simulink model "Controllo_XY"  (R2020b)
settings: Solver=VariableStepAuto  StartTime=0.0  StopTime=3  RelTol=1e-3
values from neighbouring files (symbols this model uses):
  mx = config_dc_x(parx)    [Main_Strategia_di_pilotaggio.m]    (also in Main_traiettoria.m; Main_traiettoria_ordinato.m)
  my = config_dc_y(pary)    [Main_Strategia_di_pilotaggio.m]    (also in Main_traiettoria.m; Main_traiettoria_ordinato.m)
undefined symbols (not defined in the file or in its folder): accelerazioni, accelerazioniy, Evaluate_Trajectory, parx, pary
libraries: cstblocks x8
settings Model: Creator=stefa  LastModifiedBy=user
settings DebuggingCC: SFMachineParentedDataDiag=error

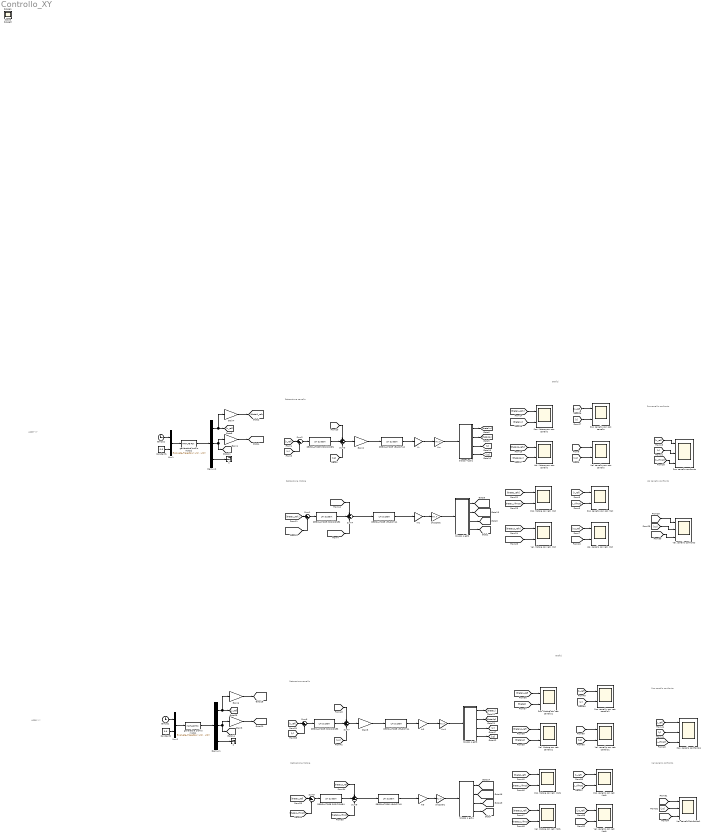
== system Controllo_XY ==
  note: ASSE "X"
  note: Retroazione carrello
  note: Retroazione Motore
  note: Grafici
  note: Pos carrello confronto
  note: Vel carrello confronto
  note: Retroazione carrello
  note: Grafici
  note: Retroazione Motore
  note: Pos carrello confronto
  note: Vel carrello confronto
  note: ASSE "Y"
  " 1" : Terminator
  " 2" : Terminator
  Constant1 : Constant  Value=0.6
  Constant2 : Constant  Value=0.6
  Demux1 : Demux  Outputs=3
  Demux2 : Demux  Outputs=3
  Gain1 : Gain  Gain=1/parx.tau
  Gain2 : Gain  Gain=1/parx.tau
  Gain3 : Gain  Gain=1/pary.tau
  Gain4 : Gain  Gain=1/parx.tau
  Gain5 : Gain  Gain=1/pary.tau
  Gain6 : Gain  Gain=1/pary.tau
  Km : Gain  Gain=mx.K
  Km1 : Gain  Gain=my.K
  Kr : Gain  Gain=mx.Kr
  Kr1 : Gain  Gain=mx.Kr
  Kr2 : Gain  Gain=my.Kr
  Kr3 : Gain  Gain=my.Kr
  Mux1 : Mux  Inputs=2
  Mux2 : Mux  Inputs=2
  Pos. Motore con retr. Mot : Scope  NumInputPorts=2
  Pos. Motore con retr. Mot1 : Scope  NumInputPorts=2
  Pos. Motore con retr. carrello : Scope  NumInputPorts=2
  Pos. Motore con retr. carrello1 : Scope  NumInputPorts=2
  Pos. carrello con retr. Mot : Scope  NumInputPorts=2
  Pos. carrello con retr. Mot1 : Scope  NumInputPorts=2
  Pos. carrello con retr. carrello : Scope  NumInputPorts=2
  Pos. carrello con retr. carrello1 : Scope  NumInputPorts=2
  Pos. carrello confronto : Scope  NumInputPorts=3
  Pos. carrello confronto1 : Scope  NumInputPorts=3
  REGOLATORE POSIZIONE1 : cstblocks/LTI System  sys=apx.H_P  IC=[]
  REGOLATORE POSIZIONE2 : cstblocks/LTI System  sys=apx.H_P  IC=[]
  REGOLATORE POSIZIONE3 : cstblocks/LTI System  sys=apy.H_P  IC=[]
  REGOLATORE POSIZIONE4 : cstblocks/LTI System  sys=apy.H_P  IC=[]
  REGOLATORE VELOCITA1 : cstblocks/LTI System  sys=avx.PI_V  IC=[]
  REGOLATORE VELOCITA2 : cstblocks/LTI System  sys=avx.PI_V  IC=[]
  REGOLATORE VELOCITA3 : cstblocks/LTI System  sys=avy.PI_V  IC=[]
  REGOLATORE VELOCITA4 : cstblocks/LTI System  sys=avy.PI_V  IC=[]
  Sum{1..2,5..6} (4 alike) : Sum  Inputs=|+-
  Sum{3..4,7..8} (4 alike) : Sum  Inputs=++-
  Vel. Motore con retr. Mot : Scope  NumInputPorts=2
  Vel. Motore con retr. Mot1 : Scope  NumInputPorts=2
  Vel. Motore con retr. carrello : Scope  NumInputPorts=2
  Vel. Motore con retr. carrello1 : Scope  NumInputPorts=2
  Vel. carrello con retr. Mot : Scope  NumInputPorts=2
  Vel. carrello con retr. Mot1 : Scope  NumInputPorts=2
  Vel. carrello con retr. carrello : Scope  NumInputPorts=2
  Vel. carrello con retr. carrello1 : Scope  NumInputPorts=2
  Vel. carrello confronto : Scope  NumInputPorts=3
  Vel. carrello confronto1 : Scope  NumInputPorts=3
  blocco 4 gdl1 : Subsystem
  blocco 4 gdl2 : Subsystem
  blocco 4 gdl3 : Subsystem
  blocco 4 gdl4 : Subsystem
  chopper1 : Gain  Gain=my.K
  chopper2 : Gain  Gain=mx.K
  generatore profilo moto1 : MATLABFcn  MATLABFcn=Evaluate_Trajectory( u(1) , u(2))  OutputDimensions=3
  generatore profilo moto2 : MATLABFcn  MATLABFcn=Evaluate_Trajectory( u(1) , u(2))  OutputDimensions=3
  tempo1 : Clock
  tempo2 : Clock
  Scope : Scope
  Scope1 : Scope
  Scope3 : Scope
  wires:
  Kr/1 -> Km/1  "I"
  REGOLATORE VELOCITA2/1 -> Kr/1  "Va"
  REGOLATORE POSIZIONE1/1 -> Sum3/2
  Demux2/3 -> " 1"/1  "XPP"
  Mux1/1 -> generatore profilo moto2/1
  generatore profilo moto2/1 -> Demux2/1  "carrello"
  Constant1/1 -> Mux1/2
  [xp_ref] -> Vel. carrello con retr. carrello/1  "xp_ref"
  [xp] -> Vel. carrello con retr. carrello/2  "xp"
  [x_ref] -> Pos. carrello con retr. carrello/1  "x_ref"
  [x] -> Pos. carrello con retr. carrello/2  "x"
  Sum2/1 -> REGOLATORE POSIZIONE1/1
  tempo2/1 -> Mux1/1
  Demux2/1 -> [x_ref], Gain4/1  "X"
  Demux2/2 -> Gain1/1, [xp_ref]  "XP"
  [xp_ref] -> Sum3/1
  Sum3/1 -> Gain2/1
  Gain2/1 -> REGOLATORE VELOCITA2/1  "theta1_rifx"
  [x_ref] -> Sum2/1
  [x] -> Sum2/2
  [xp] -> Sum3/3
  [x_rifmot] -> Pos. carrello con retr. Mot/2  "x_rif"
  [theta1_refx] -> Pos. Motore con retr. Mot/1  "theta1_ref"
  Kr1/1 -> chopper2/1  "I"
  Sum1/1 -> REGOLATORE POSIZIONE2/1
  [theta1p_refx] -> Vel. Motore con retr. Mot/1  "theta1p_ref"
  REGOLATORE POSIZIONE2/1 -> Sum4/2
  REGOLATORE VELOCITA1/1 -> Kr1/1  "Va"
  [xp_rifmot] -> Vel. carrello con retr. Mot/2  "xp"
  [xp_ref] -> Vel. carrello con retr. Mot/1  "xp_ref"
  Sum4/1 -> REGOLATORE VELOCITA1/1
  [x_ref] -> Pos. carrello con retr. Mot/1  "x"
  [theta1p_rifmotx] -> Vel. Motore con retr. Mot/2  "theta1p"
  [theta1_rifmotx] -> Pos. Motore con retr. Mot/2  "theta1"
  [theta1p_refx] -> Sum4/1
  [theta1_refx] -> Sum1/1
  [theta1p_rifmotx] -> Sum4/3
  [theta1_rifmotx] -> Sum1/2
  [theta1px] -> Vel. Motore con retr. carrello/2  "thehta1p"
  [theta1x] -> Pos. Motore con retr. carrello/2  "tetha1"
  [theta1p_refx] -> Vel. Motore con retr. carrello/1  "theta1p_ref"
  [theta1_refx] -> Pos. Motore con retr. carrello/1  "theta1_ref"
  [x] -> Pos. carrello confronto/2  "x_retcarr"
  [x_ref] -> Pos. carrello confronto/1  "x_ref"
  [x_rifmot] -> Pos. carrello confronto/3  "x_retmot"
  [xp] -> Vel. carrello confronto/2  "xp_retcarr"
  [xp_ref] -> Vel. carrello confronto/1  "xp_ref"
  [xp_rifmot] -> Vel. carrello confronto/3  "xp_retmot"
  Km/1 -> blocco 4 gdl1/1(In1)  "Cm"
  Gain1/1 -> [theta1p_refx]  "motore"
  Gain4/1 -> [theta1_refx]  "motore"
  chopper2/1 -> blocco 4 gdl2/1(In1)  "Cm"
  blocco 4 gdl1/1(Out3) -> [theta1x]
  blocco 4 gdl1/2(Out4) -> [theta1px]
  blocco 4 gdl1/3(Out7) -> [x]
  blocco 4 gdl1/4(Out8) -> [xp]
  blocco 4 gdl2/1(Out3) -> [theta1_rifmotx]
  blocco 4 gdl2/3(Out7) -> [x_rifmot]
  blocco 4 gdl2/2(Out4) -> [theta1p_rifmotx]
  blocco 4 gdl2/4(Out1) -> [xp_rifmot]
  [yp] -> Sum7/3
  Kr3/1 -> chopper1/1  "I"
  [yp_ref] -> Vel. carrello confronto1/1  "yp ldm"
  Demux1/1 -> [y_ref], Gain6/1  "Y"
  [y_rifmot] -> Pos. carrello confronto1/3  "y retr. motore"
  chopper1/1 -> blocco 4 gdl4/1(In1)  "Cm"
  [y_ref] -> Pos. carrello con retr. Mot1/1  "y_ref"
  blocco 4 gdl3/4(Out4) -> [yp]
  [theta1p_ref] -> Vel. Motore con retr. carrello1/1  "thehta1p_ref"
  Gain5/1 -> REGOLATORE VELOCITA4/1  "theta1_rif"
  [theta1p] -> Vel. Motore con retr. carrello1/2  "theta1p"
  tempo1/1 -> Mux2/1
  [theta1] -> Pos. Motore con retr. carrello1/2  "theta1"
  [y] -> Pos. carrello confronto1/2  "y retr. carrello"
  blocco 4 gdl4/2(Out1) -> [theta1p_rifmot]
  [theta1_ref] -> Pos. Motore con retr. Mot1/1  "theta1_ref"
  [theta1_ref] -> Sum5/1
  Gain6/1 -> [theta1_ref]  "motore"
  [theta1p_rifmot] -> Vel. Motore con retr. Mot1/2  "theta1p"
  blocco 4 gdl4/1(Out2) -> [theta1_rifmot]
  [yp] -> Vel. carrello con retr. carrello1/2  "yp"
  [y_rifmot] -> Pos. carrello con retr. Mot1/2  "y"
  Sum7/1 -> Gain5/1
  [theta1p_ref] -> Sum8/1
  Gain3/1 -> [theta1p_ref]  "motore"
  Sum8/1 -> REGOLATORE VELOCITA3/1
  [yp] -> Vel. carrello confronto1/2
  Demux1/3 -> " 2"/1  "YPP"
  [yp_rifmot] -> Vel. carrello con retr. Mot1/2  "yp"
  [yp_rifmot] -> Vel. carrello confronto1/3
  [theta1p_ref] -> Vel. Motore con retr. Mot1/1  "thehta1p_ref"
  REGOLATORE VELOCITA3/1 -> Kr3/1  "Va"
  [y] -> Sum6/2
  [theta1_ref] -> Pos. Motore con retr. carrello1/1  "theta1_ref"
  Demux1/2 -> Gain3/1, [yp_ref]  "YP"
  Sum6/1 -> REGOLATORE POSIZIONE3/1
  [theta1_rifmot] -> Sum5/2
  [y_ref] -> Sum6/1
  REGOLATORE VELOCITA4/1 -> Kr2/1  "Va"
  [yp_ref] -> Vel. carrello con retr. carrello1/1  "yp_ref"
  generatore profilo moto1/1 -> Demux1/1  "carrello"
  blocco 4 gdl4/4(Out4) -> [yp_rifmot]
  [theta1p_rifmot] -> Sum8/3
  blocco 4 gdl3/1(Out2) -> [theta1]
  [y] -> Pos. carrello con retr. carrello1/2  "y"
  [yp_ref] -> Vel. carrello con retr. Mot1/1  "yp_ref"
  Sum5/1 -> REGOLATORE POSIZIONE4/1
  [y_ref] -> Pos. carrello con retr. carrello1/1  "y_ref"
  [yp_ref] -> Sum7/1
  REGOLATORE POSIZIONE4/1 -> Sum8/2
  Km1/1 -> blocco 4 gdl3/1(In1)  "Cm"
  blocco 4 gdl3/3(Out3) -> [y]
  [y_ref] -> Pos. carrello confronto1/1  "y ldm"
  Mux2/1 -> generatore profilo moto1/1
  REGOLATORE POSIZIONE3/1 -> Sum7/2
  Constant2/1 -> Mux2/2
  [theta1_rifmot] -> Pos. Motore con retr. Mot1/2  "theta1"
  Kr2/1 -> Km1/1  "I"
  blocco 4 gdl3/2(Out1) -> [theta1p]
  blocco 4 gdl4/3(Out3) -> [y_rifmot]

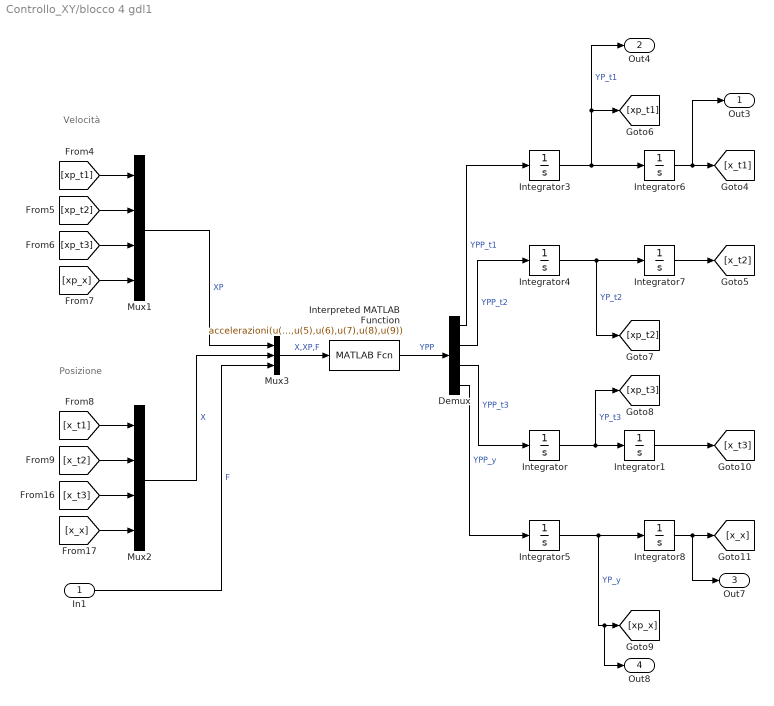
== system Controllo_XY/blocco 4 gdl1 ==
  note: Velocità
  note: Posizione
  In1 : Inport
  Demux : Demux
  Integrator{,1,3..7} (7 alike) : Integrator
  Integrator8 : Integrator  InitialCondition=0.0005
  Interpreted MATLAB Function : MATLABFcn  MATLABFcn=accelerazioni(u(1),u(2),u(3),u(4),u(5),u(6),u(7),u(8),u(9))  OutputDimensions=4
  Mux1 : Mux
  Mux2 : Mux
  Mux3 : Mux  Inputs=3
  Out3 : Outport
  Out4 : Outport  Port=2
  Out7 : Outport  Port=3
  Out8 : Outport  Port=4
  wires:
  Integrator4/1 -> [xp_t2], Integrator7/1  "YP_t2"
  [xp_t1] -> Mux1/1
  [x_t2] -> Mux2/2
  Integrator1/1 -> [x_t3]
  Demux/4 -> Integrator5/1  "YPP_y"
  Demux/2 -> Integrator4/1  "YPP_t2"
  In1/1 -> Mux3/3  "F"
  Mux3/1 -> Interpreted MATLAB Function/1  "X,XP,F"
  [xp_t2] -> Mux1/2
  Integrator6/1 -> Out3/1, [x_t1]
  Mux2/1 -> Mux3/2  "X"
  Demux/3 -> Integrator/1  "YPP_t3"
  Integrator5/1 -> Out8/1, [xp_x], Integrator8/1  "YP_y"
  Integrator8/1 -> Out7/1, [x_x]
  [xp_x] -> Mux1/4
  [x_x] -> Mux2/4
  Integrator7/1 -> [x_t2]
  Demux/1 -> Integrator3/1  "YPP_t1"
  [x_t1] -> Mux2/1
  Integrator3/1 -> Out4/1, [xp_t1], Integrator6/1  "YP_t1"
  [x_t3] -> Mux2/3
  Interpreted MATLAB Function/1 -> Demux/1  "YPP"
  Mux1/1 -> Mux3/1  "XP"
  Integrator/1 -> Integrator1/1, [xp_t3]  "YP_t3"
  [xp_t3] -> Mux1/3

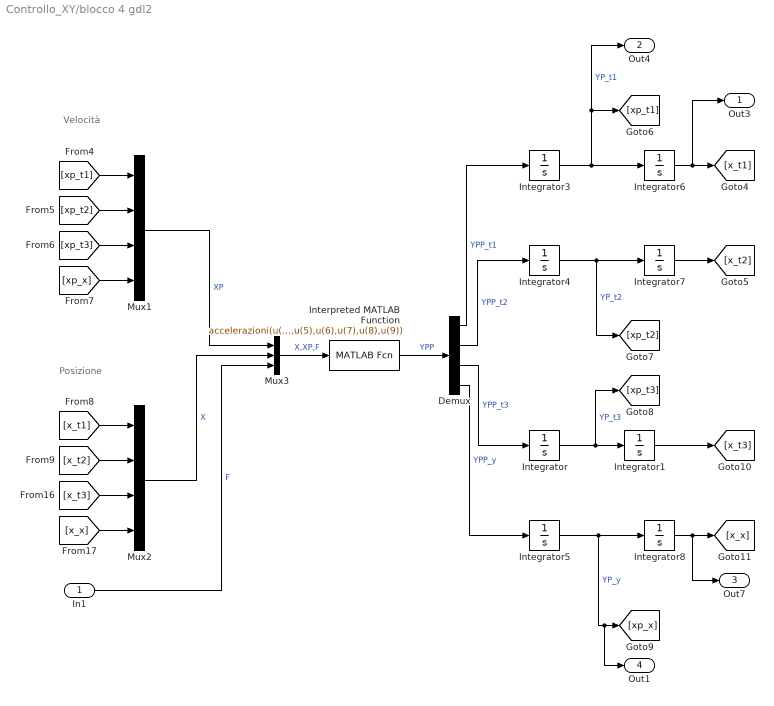
== system Controllo_XY/blocco 4 gdl2 ==
  note: Posizione
  note: Velocità
  In1 : Inport
  Demux : Demux
  Integrator{,1,3..7} (7 alike) : Integrator
  Integrator8 : Integrator  InitialCondition=0.0005
  Interpreted MATLAB Function : MATLABFcn  MATLABFcn=accelerazioni(u(1),u(2),u(3),u(4),u(5),u(6),u(7),u(8),u(9))  OutputDimensions=4
  Mux1 : Mux
  Mux2 : Mux
  Mux3 : Mux  Inputs=3
  Out3 : Outport
  Out4 : Outport  Port=2
  Out7 : Outport  Port=3
  Out1 : Outport  Port=4
  wires:
  [xp_t3] -> Mux1/3
  Interpreted MATLAB Function/1 -> Demux/1  "YPP"
  Integrator3/1 -> Out4/1, [xp_t1], Integrator6/1  "YP_t1"
  Integrator8/1 -> Out7/1, [x_x]
  Integrator7/1 -> [x_t2]
  [xp_x] -> Mux1/4
  [x_t1] -> Mux2/1
  Mux1/1 -> Mux3/1  "XP"
  [x_x] -> Mux2/4
  Demux/3 -> Integrator/1  "YPP_t3"
  Integrator/1 -> Integrator1/1, [xp_t3]  "YP_t3"
  Mux2/1 -> Mux3/2  "X"
  Integrator6/1 -> Out3/1, [x_t1]
  Integrator5/1 -> Out1/1, [xp_x], Integrator8/1  "YP_y"
  [xp_t2] -> Mux1/2
  Mux3/1 -> Interpreted MATLAB Function/1  "X,XP,F"
  [x_t3] -> Mux2/3
  In1/1 -> Mux3/3  "F"
  Demux/4 -> Integrator5/1  "YPP_y"
  Integrator4/1 -> [xp_t2], Integrator7/1  "YP_t2"
  Integrator1/1 -> [x_t3]
  [xp_t1] -> Mux1/1
  [x_t2] -> Mux2/2
  Demux/2 -> Integrator4/1  "YPP_t2"
  Demux/1 -> Integrator3/1  "YPP_t1"

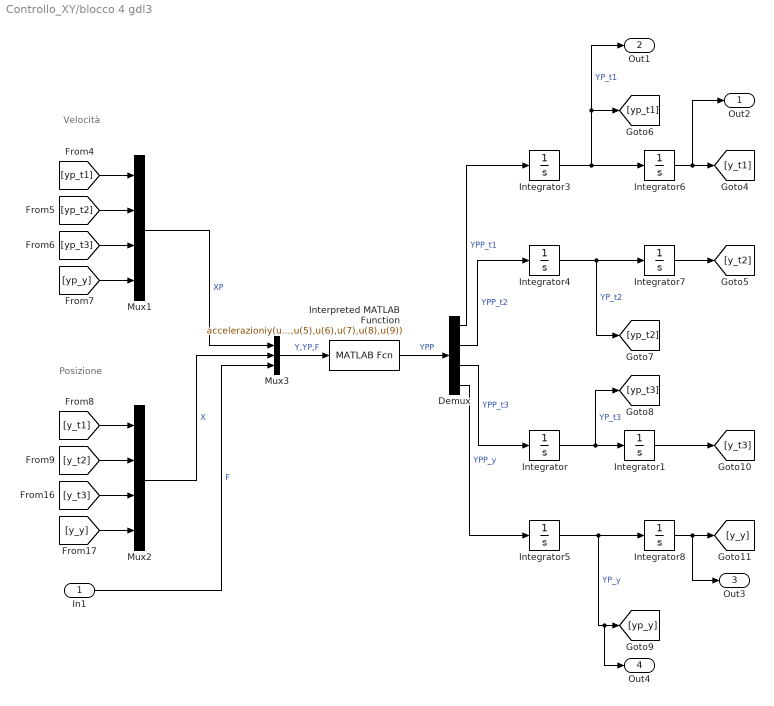
== system Controllo_XY/blocco 4 gdl3 ==
  note: Posizione
  note: Velocità
  In1 : Inport
  Demux : Demux
  Integrator{,1,3..7} (7 alike) : Integrator
  Integrator8 : Integrator  InitialCondition=0.0005
  Interpreted MATLAB Function : MATLABFcn  MATLABFcn=accelerazioniy(u(1),u(2),u(3),u(4),u(5),u(6),u(7),u(8),u(9))  OutputDimensions=4
  Mux1 : Mux
  Mux2 : Mux
  Mux3 : Mux  Inputs=3
  Out2 : Outport
  Out1 : Outport  Port=2
  Out3 : Outport  Port=3
  Out4 : Outport  Port=4
  wires:
  Integrator/1 -> Integrator1/1, [yp_t3]  "YP_t3"
  Mux1/1 -> Mux3/1  "XP"
  [y_t3] -> Mux2/3
  Mux3/1 -> Interpreted MATLAB Function/1  "Y,YP,F"
  [y_t2] -> Mux2/2
  Integrator7/1 -> [y_t2]
  Demux/3 -> Integrator/1  "YPP_t3"
  [yp_y] -> Mux1/4
  [y_y] -> Mux2/4
  Demux/1 -> Integrator3/1  "YPP_t1"
  [yp_t2] -> Mux1/2
  Mux2/1 -> Mux3/2  "X"
  Interpreted MATLAB Function/1 -> Demux/1  "YPP"
  Integrator8/1 -> Out3/1, [y_y]
  Integrator4/1 -> [yp_t2], Integrator7/1  "YP_t2"
  Integrator3/1 -> Out1/1, [yp_t1], Integrator6/1  "YP_t1"
  In1/1 -> Mux3/3  "F"
  Demux/2 -> Integrator4/1  "YPP_t2"
  Integrator5/1 -> Out4/1, [yp_y], Integrator8/1  "YP_y"
  Integrator6/1 -> Out2/1, [y_t1]
  [yp_t3] -> Mux1/3
  Demux/4 -> Integrator5/1  "YPP_y"
  Integrator1/1 -> [y_t3]
  [yp_t1] -> Mux1/1
  [y_t1] -> Mux2/1

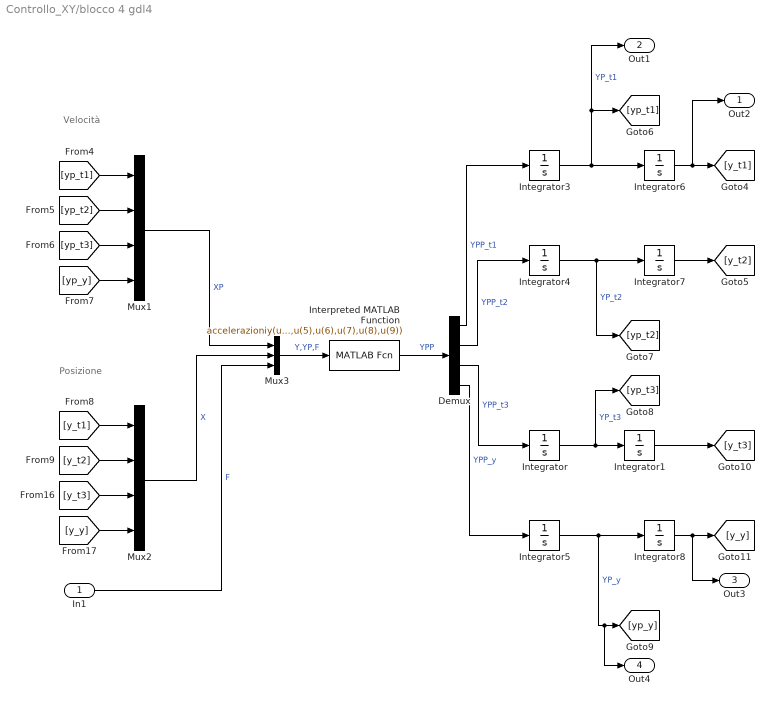
== system Controllo_XY/blocco 4 gdl4 ==
  note: Posizione
  note: Velocità
  In1 : Inport
  Demux : Demux
  Integrator{,1,3..7} (7 alike) : Integrator
  Integrator8 : Integrator  InitialCondition=0.0005
  Interpreted MATLAB Function : MATLABFcn  MATLABFcn=accelerazioniy(u(1),u(2),u(3),u(4),u(5),u(6),u(7),u(8),u(9))  OutputDimensions=4
  Mux1 : Mux
  Mux2 : Mux
  Mux3 : Mux  Inputs=3
  Out2 : Outport
  Out1 : Outport  Port=2
  Out3 : Outport  Port=3
  Out4 : Outport  Port=4
  wires:
  Integrator/1 -> Integrator1/1, [yp_t3]  "YP_t3"
  Mux1/1 -> Mux3/1  "XP"
  [y_t3] -> Mux2/3
  Mux3/1 -> Interpreted MATLAB Function/1  "Y,YP,F"
  [y_t2] -> Mux2/2
  Integrator7/1 -> [y_t2]
  Demux/3 -> Integrator/1  "YPP_t3"
  [yp_y] -> Mux1/4
  [y_y] -> Mux2/4
  Demux/1 -> Integrator3/1  "YPP_t1"
  [yp_t2] -> Mux1/2
  Mux2/1 -> Mux3/2  "X"
  Interpreted MATLAB Function/1 -> Demux/1  "YPP"
  Integrator8/1 -> Out3/1, [y_y]
  Integrator4/1 -> [yp_t2], Integrator7/1  "YP_t2"
  Integrator3/1 -> Out1/1, [yp_t1], Integrator6/1  "YP_t1"
  In1/1 -> Mux3/3  "F"
  Demux/2 -> Integrator4/1  "YPP_t2"
  Integrator5/1 -> Out4/1, [yp_y], Integrator8/1  "YP_y"
  Integrator6/1 -> Out2/1, [y_t1]
  [yp_t3] -> Mux1/3
  Demux/4 -> Integrator5/1  "YPP_y"
  Integrator1/1 -> [y_t3]
  [yp_t1] -> Mux1/1
  [y_t1] -> Mux2/1
